simulink model "AC1A"  (R2020a)
settings: Solver=ode1  StartTime=0.0  StopTime=5  FixedStep=Ts  RelTol=1e-3  EnableMultiTasking=on
undefined symbols (not defined in the file or in its folder): GABDA, GABDB, GBBDA, GBBDB, GPPMA, GPPMB, GPPMC, SADA, SADB, SADC, SADD, SBDA, SBDC, SBSB, SCDA, SCDC, SCDD, SCSB, SDDA, SDDB, SDDC, SDDD, SDDE, Ts, TsCont
libraries: simulink x5, sps_avr x2
settings Model: Creator=gdudgeon  LastModifiedBy=gdudgeon
settings SolverCC: ConcurrentTasks=on  AutoInsertRateTranBlk=on  InsertRTBMode=Never (minimum delay)
settings DataIOCC: SaveFormat=StructureWithTime  SaveOutput=off  SaveTime=off
settings OptimizationCC: BlockReduction=off  OptimizeBlockIOStorage=off  BufferReuse=off  GlobalBufferReuse=off  ExpressionFolding=off  LocalBlockOutputs=off  OptimizeDataStoreBuffers=off  BusAssignmentInplaceUpdate=off
settings HardwareCC: ProdBitPerPointer=32  ProdBitPerSizeT=32  ProdBitPerPtrDiffT=32  ProdLargestAtomicFloat=None  ProdWordSize=32  ProdLongLongMode=on  ProdHWDeviceType=Generic->32-bit x86 compatible
settings ModelReferenceCC: ModelReferenceNumInstancesAllowed=Single
settings SFSimCC: CustomCodeUndefinedFunction=UseInterfaceOnly
settings RTWCC: Description=Simulink Real-Time  SystemTargetFile=slrt.tlc  TemplateMakefile=slrt_default_tmf  CodeExecutionProfiling=on  RTWCompilerOptimization=on
settings SimulinkRealTimeCC: SupportVariableSizeSignals=on  RL32LogTETModifier=off  xPCConcurrentTasks=on

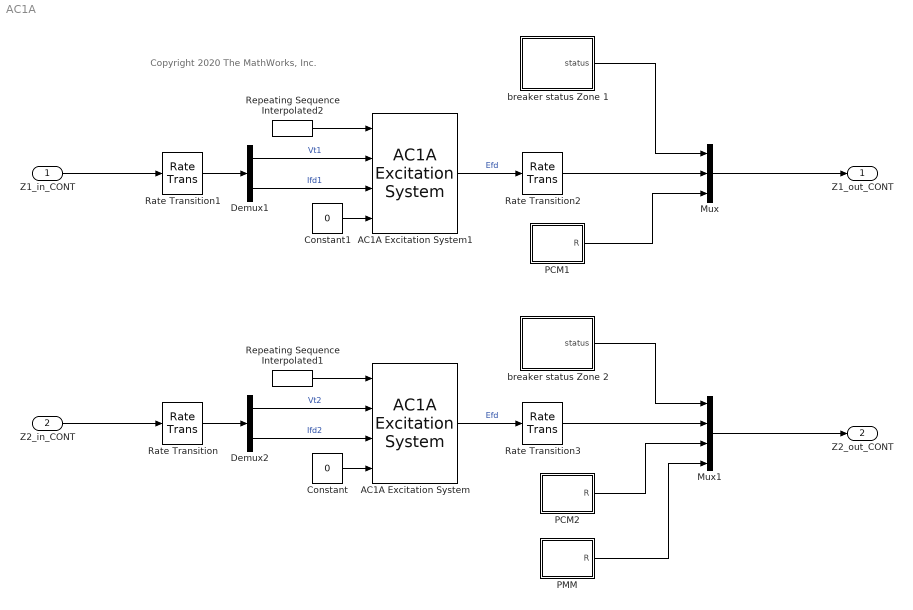
== system AC1A ==
  note: Copyright 2020 The MathWorks, Inc.
  Z1_in_CONT : Inport  OutDataTypeStr=double  PortDimensions=2  SampleTime=Ts
  Z2_in_CONT : Inport  Port=2  OutDataTypeStr=double  PortDimensions=2  SampleTime=Ts
  AC1A Excitation System : sps_avr/AC1A Excitation System  Tr=0.001  KaTa=[80 0.2]  VAminmax=[-15 15]  VRminmax=[-14.99 14.99]  KfTf=[0.03 1.49]  TbTc=[0 0]  KeTe=[1.0 0.2]  Ve12=[5 4]  SeVe12=[0.4 0.5]  Kd=0.4  Kc=1  v0=[1 1]  TsBlock=TsCont
      settings: SourceProductBaseCode=PS
  AC1A Excitation System1 : sps_avr/AC1A Excitation System  Tr=0.001  KaTa=[80 0.2]  VAminmax=[-15 15]  VRminmax=[-14.99 14.99]  KfTf=[0.03 1.49]  TbTc=[0 0]  KeTe=[1.0 0.2]  Ve12=[5 4]  SeVe12=[0.4 0.5]  Kd=0.4  Kc=1  v0=[1 1]  TsBlock=TsCont
      settings: SourceProductBaseCode=PS
  Constant : Constant  Value=0  SampleTime=TsCont
  Constant1 : Constant  Value=0  SampleTime=TsCont
  Demux1 : Demux  Outputs=2
  Demux2 : Demux  Outputs=2
  Mux : Mux  Inputs=[9 1 1]
  Mux1 : Mux  Inputs=[14 1 1 1]
  PCM1 : Subsystem
  PCM2 : Subsystem
  PMM : Subsystem
  Rate Transition : RateTransition  Deterministic=off  OutPortSampleTime=TsCont
  Rate Transition1 : RateTransition  Deterministic=off  OutPortSampleTime=TsCont
  Rate Transition2 : RateTransition  Deterministic=off  OutPortSampleTime=Ts
  Rate Transition3 : RateTransition  Deterministic=off  OutPortSampleTime=Ts
  Repeating Sequence Interpolated1 : simulink/Sources/Repeating Sequence Interpolated  OutValues=[1 1 1]  TimeValues=[0 5 1000]  LookUpMeth=Interpolation-Use End Values  tsamp=TsCont  OutMin=[]  OutMax=[]  OutDataTypeStr=double  OutputDataTypeScalingMode=double  OutDataType=fixdt(0,8)  OutScaling=2^-10
  Repeating Sequence Interpolated2 : simulink/Sources/Repeating Sequence Interpolated  OutValues=[1 1 1]  TimeValues=[0 5 1000]  LookUpMeth=Interpolation-Use End Values  tsamp=TsCont  OutMin=[]  OutMax=[]  OutDataTypeStr=double  OutputDataTypeScalingMode=double  OutDataType=fixdt(0,8)  OutScaling=2^-10
  breaker status Zone 1 : Subsystem
  breaker status Zone 2 : Subsystem
  Z1_out_CONT : Outport  PortDimensions=11  SampleTime=Ts  VectorParamsAs1DForOutWhenUnconnected=off
  Z2_out_CONT : Outport  Port=2  PortDimensions=17  SampleTime=Ts  VectorParamsAs1DForOutWhenUnconnected=off
  wires:
  Z2_in_CONT/1 -> Rate Transition/1
  Rate Transition/1 -> Demux2/1
  Repeating Sequence Interpolated1/1 -> AC1A Excitation System/1
  Demux2/1 -> AC1A Excitation System/2  "Vt2"
  Demux2/2 -> AC1A Excitation System/3  "Ifd2"
  Constant/1 -> AC1A Excitation System/4
  breaker status Zone 2/1(status) -> Mux1/1
  AC1A Excitation System/1 -> Rate Transition3/1  "Efd"
  PCM2/1(R) -> Mux1/3
  PMM/1(R) -> Mux1/4
  AC1A Excitation System1/1 -> Rate Transition2/1  "Efd"
  Constant1/1 -> AC1A Excitation System1/4
  Demux1/2 -> AC1A Excitation System1/3  "Ifd1"
  Demux1/1 -> AC1A Excitation System1/2  "Vt1"
  Repeating Sequence Interpolated2/1 -> AC1A Excitation System1/1
  Rate Transition1/1 -> Demux1/1
  Z1_in_CONT/1 -> Rate Transition1/1
  PCM1/1(R) -> Mux/3
  breaker status Zone 1/1(status) -> Mux/1
  Rate Transition2/1 -> Mux/2
  Rate Transition3/1 -> Mux1/2
  Mux/1 -> Z1_out_CONT/1
  Mux1/1 -> Z2_out_CONT/1

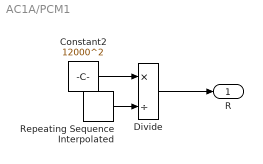
== system AC1A/PCM1 ==
  Constant2 : Constant  Value=12000^2  SampleTime=Ts
  Divide : Product  Inputs=*/
  Repeating Sequence Interpolated : simulink/Sources/Repeating Sequence Interpolated  OutValues=[1e3 1e3 10e6 10e6].'  TimeValues=[0 10 20 100].'  LookUpMeth=Interpolation-Use End Values  tsamp=Ts  OutMin=[]  OutMax=[]  OutDataTypeStr=double  OutputDataTypeScalingMode=double  OutDataType=fixdt(0,8)  OutScaling=2^-10
  R : Outport  VectorParamsAs1DForOutWhenUnconnected=off
  wires:
  Constant2/1 -> Divide/1
  Repeating Sequence Interpolated/1 -> Divide/2
  Divide/1 -> R/1

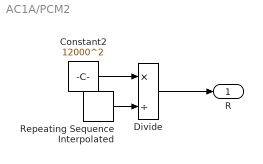
== system AC1A/PCM2 ==
  Constant2 : Constant  Value=12000^2  SampleTime=Ts
  Divide : Product  Inputs=*/
  Repeating Sequence Interpolated : simulink/Sources/Repeating Sequence Interpolated  OutValues=[1e3 1e3 10e6 10e6].'  TimeValues=[0 15 20 100].'  LookUpMeth=Interpolation-Use End Values  tsamp=Ts  OutMin=[]  OutMax=[]  OutDataTypeStr=double  OutputDataTypeScalingMode=double  OutDataType=fixdt(0,8)  OutScaling=2^-10
  R : Outport  VectorParamsAs1DForOutWhenUnconnected=off
  wires:
  Divide/1 -> R/1
  Repeating Sequence Interpolated/1 -> Divide/2
  Constant2/1 -> Divide/1

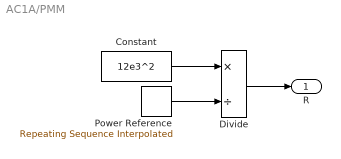
== system AC1A/PMM ==
  Constant : Constant  Value=12e3^2  SampleTime=Ts
  Divide : Product  Inputs=*/
  Power Reference : simulink/Sources/Repeating Sequence Interpolated  OutValues=[1 1 1 1]*8.4e6  TimeValues=[0 7 12 100]  LookUpMeth=Interpolation-Use End Values  tsamp=Ts  OutMin=[]  OutMax=[]  OutDataTypeStr=double  OutputDataTypeScalingMode=double  OutDataType=fixdt(0,8)  OutScaling=2^-10
  R : Outport  VectorParamsAs1DForOutWhenUnconnected=off
  wires:
  Divide/1 -> R/1
  Constant/1 -> Divide/1
  Power Reference/1 -> Divide/2

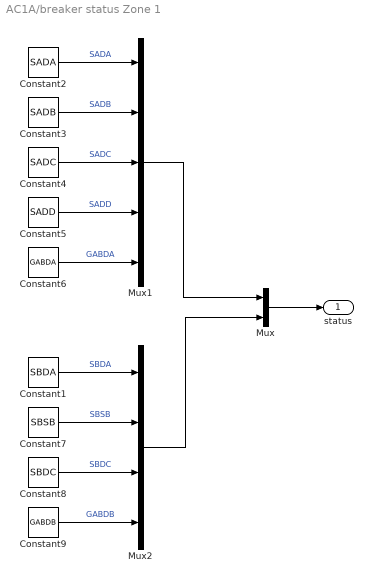
== system AC1A/breaker status Zone 1 ==
  Constant1 : Constant  Value=SBDA  SampleTime=Ts
  Constant2 : Constant  Value=SADA  SampleTime=Ts
  Constant3 : Constant  Value=SADB  SampleTime=Ts
  Constant4 : Constant  Value=SADC  SampleTime=Ts
  Constant5 : Constant  Value=SADD  SampleTime=Ts
  Constant6 : Constant  Value=GABDA  SampleTime=Ts
  Constant7 : Constant  Value=SBSB  SampleTime=Ts
  Constant8 : Constant  Value=SBDC  SampleTime=Ts
  Constant9 : Constant  Value=GABDB  SampleTime=Ts
  Mux : Mux  Inputs=[5 4]
  Mux1 : Mux  Inputs=5
  Mux2 : Mux
  status : Outport  VectorParamsAs1DForOutWhenUnconnected=off
  wires:
  Constant5/1 -> Mux1/4  "SADD"
  Constant2/1 -> Mux1/1  "SADA"
  Constant3/1 -> Mux1/2  "SADB"
  Constant4/1 -> Mux1/3  "SADC"
  Constant6/1 -> Mux1/5  "GABDA"
  Constant1/1 -> Mux2/1  "SBDA"
  Constant7/1 -> Mux2/2  "SBSB"
  Constant8/1 -> Mux2/3  "SBDC"
  Constant9/1 -> Mux2/4  "GABDB"
  Mux/1 -> status/1
  Mux1/1 -> Mux/1
  Mux2/1 -> Mux/2

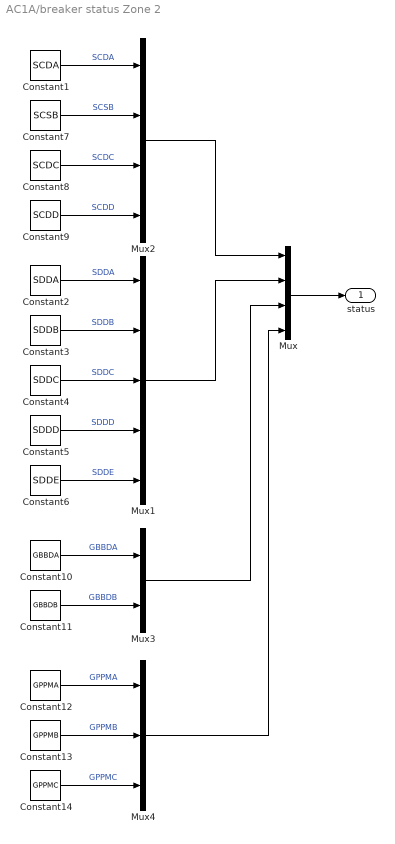
== system AC1A/breaker status Zone 2 ==
  Constant1 : Constant  Value=SCDA  SampleTime=Ts
  Constant10 : Constant  Value=GBBDA  SampleTime=Ts
  Constant11 : Constant  Value=GBBDB  SampleTime=Ts
  Constant12 : Constant  Value=GPPMA  SampleTime=Ts
  Constant13 : Constant  Value=GPPMB  SampleTime=Ts
  Constant14 : Constant  Value=GPPMC  SampleTime=Ts
  Constant2 : Constant  Value=SDDA  SampleTime=Ts
  Constant3 : Constant  Value=SDDB  SampleTime=Ts
  Constant4 : Constant  Value=SDDC  SampleTime=Ts
  Constant5 : Constant  Value=SDDD  SampleTime=Ts
  Constant6 : Constant  Value=SDDE  SampleTime=Ts
  Constant7 : Constant  Value=SCSB  SampleTime=Ts
  Constant8 : Constant  Value=SCDC  SampleTime=Ts
  Constant9 : Constant  Value=SCDD  SampleTime=Ts
  Mux : Mux  Inputs=[4 5 2 3]
  Mux1 : Mux  Inputs=5
  Mux2 : Mux
  Mux3 : Mux  Inputs=2
  Mux4 : Mux  Inputs=3
  status : Outport  VectorParamsAs1DForOutWhenUnconnected=off
  wires:
  Mux/1 -> status/1
  Constant9/1 -> Mux2/4  "SCDD"
  Constant8/1 -> Mux2/3  "SCDC"
  Constant7/1 -> Mux2/2  "SCSB"
  Constant1/1 -> Mux2/1  "SCDA"
  Constant6/1 -> Mux1/5  "SDDE"
  Constant4/1 -> Mux1/3  "SDDC"
  Constant3/1 -> Mux1/2  "SDDB"
  Constant2/1 -> Mux1/1  "SDDA"
  Constant5/1 -> Mux1/4  "SDDD"
  Constant10/1 -> Mux3/1  "GBBDA"
  Constant11/1 -> Mux3/2  "GBBDB"
  Constant12/1 -> Mux4/1  "GPPMA"
  Constant13/1 -> Mux4/2  "GPPMB"
  Constant14/1 -> Mux4/3  "GPPMC"
  Mux2/1 -> Mux/1
  Mux1/1 -> Mux/2
  Mux3/1 -> Mux/3
  Mux4/1 -> Mux/4
